simulink subsystem "MPC13_nlpsol"  (R2022b)
settings: Solver=VariableStepAuto  StartTime=0.0  StopTime=10.0  RelTol=1e-3
undefined symbols (not defined in the file): param_global, param_jointspace_ct, param_MPC10, param_MPC13, param_robot, param_traj, param_weight_init
settings Model: Creator=emu  LastModifiedBy=emu
settings OptimizationCC: ReuseModelBlockBuffer=on

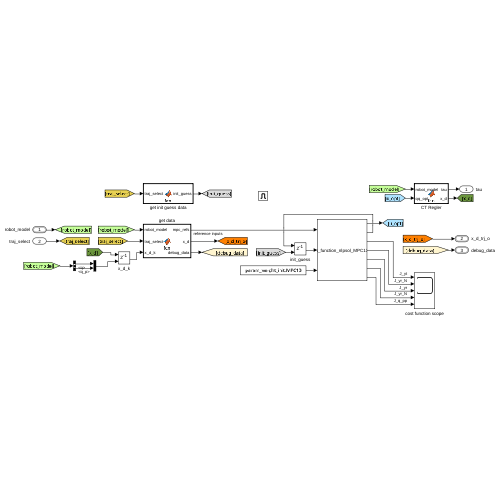
[thumbnail: Simulink's stored preview of the top-level diagram]
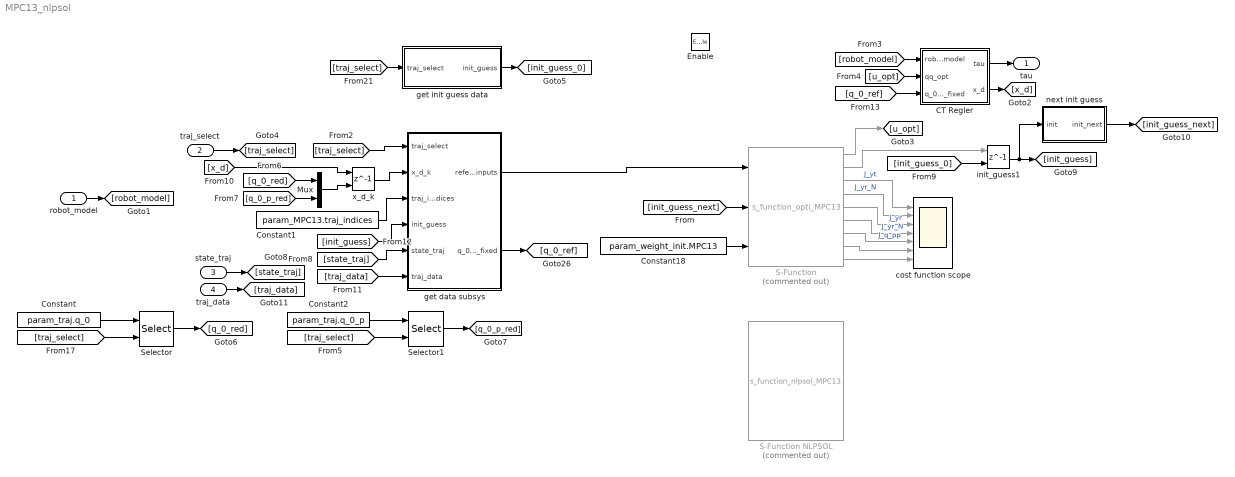
== system MPC13_nlpsol ==
  robot_model : Inport  OutDataTypeStr=Bus: robot_model
  traj_select : Inport  Port=2
  state_traj : Inport  Port=3  OutDataTypeStr=Bus: state_traj_bus
  traj_data : Inport  Port=4  OutDataTypeStr=Bus: traj_data_bus
  Enable : EnablePort
  CT Regler : MATLAB Function  TreatAsAtomicUnit=on
  Constant : Constant  Value=param_traj.q_0
  Constant1 : Constant  Value=param_MPC13.traj_indices
  Constant18 : Constant  Value=param_weight_init.MPC13  VectorParams1D=off
  Constant2 : Constant  Value=param_traj.q_0_p
  Mux : Mux  Inputs=2
  S-Function : S-Function  Commented=on  FunctionName=s_function_opti_MPC13  SFunctionModules='MPC13'  SFunctionDeploymentMode=off  EnableBusSupport=off
  S-Function NLPSOL : S-Function  Commented=on  FunctionName=s_function_nlpsol_MPC13  Parameters='s_functions/fr3_no_hand_6dof/MPC13.casadi', 'MPC13'  SFunctionModules='MPC13'  SFunctionDeploymentMode=off  EnableBusSupport=off
  Selector : Selector  NumberOfDimensions=2  InputPortWidth=3  IndexOptions=Index vector (dialog),Index vector (port)  Indices=param_robot.n_indices,1  OutputSizes=1,1
  Selector1 : Selector  NumberOfDimensions=2  InputPortWidth=3  IndexOptions=Index vector (dialog),Index vector (port)  Indices=param_robot.n_indices,1  OutputSizes=1,1
  cost function scope : Scope  NumInputPorts=7
  get data subsys : Subsystem
  get init guess data : MATLAB Function  TreatAsAtomicUnit=on
  init_guess1 : Delay  DelayLength=1  InitialConditionSource=Input port  InitialCondition=1  SampleTime=param_global.Ta
      settings: InputPortMap=u0,p4
  next init guess : MATLAB Function  TreatAsAtomicUnit=on
  x_d_k : Delay  DelayLength=1  InitialConditionSource=Input port  InitialCondition=1
      settings: InputPortMap=u0,p4
  tau : Outport
  wires:
  [init_guess_next] -> S-Function/2
  init_guess1/1 -> next init guess/1(init), [init_guess]
  next init guess/1(init_next) -> [init_guess_next]
  [state_traj] -> get data subsys/5(state_traj)
  S-Function/7 -> cost function scope/5  "J_q_pp"
  Mux/1 -> x_d_k/2
  [traj_select] -> get data subsys/1(traj_select)
  [robot_model] -> CT Regler/1(robot_model)
  Constant18/1 -> S-Function/3
  get data subsys/1(reference inputs) -> S-Function/1
  [q_0_p_red] -> Mux/2
  [traj_select] -> Selector1/2
  S-Function/8 -> cost function scope/6
  S-Function/6 -> cost function scope/4  "J_yr_N"
  [init_guess_0] -> init_guess1/2
  S-Function/5 -> cost function scope/3  "J_yr"
  get data subsys/2(q_0_ref_fixed) -> [q_0_ref]
  state_traj/1 -> [state_traj]
  [init_guess] -> get data subsys/4(init_guess)
  [q_0_red] -> Mux/1
  x_d_k/1 -> get data subsys/2(x_d_k)
  Selector/1 -> [q_0_red]
  [traj_select] -> get init guess data/1(traj_select)
  S-Function/1 -> [u_opt]
  [q_0_ref] -> CT Regler/3(q_0_ref_fixed)
  get init guess data/1(init_guess) -> [init_guess_0]
  robot_model/1 -> [robot_model]
  [traj_select] -> Selector/2
  Constant/1 -> Selector/1
  Constant2/1 -> Selector1/1
  Selector1/1 -> [q_0_p_red]
  [x_d] -> x_d_k/1
  CT Regler/1(tau) -> tau/1
  S-Function/9 -> cost function scope/7
  S-Function/4 -> cost function scope/2  "J_yr_N"
  S-Function/2 -> init_guess1/1
  Constant1/1 -> get data subsys/3(traj_indices)
  [u_opt] -> CT Regler/2(qq_opt)
  traj_select/1 -> [traj_select]
  S-Function/3 -> cost function scope/1  "J_yt"
  CT Regler/2(x_d) -> [x_d]
  traj_data/1 -> [traj_data]
  [traj_data] -> get data subsys/6(traj_data)

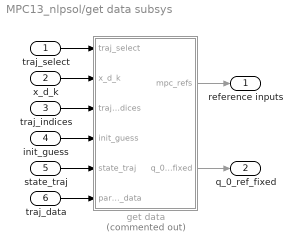
== system MPC13_nlpsol/get data subsys ==
  traj_select : Inport
  x_d_k : Inport  Port=2
  traj_indices : Inport  Port=3
  init_guess : Inport  Port=4
  state_traj : Inport  Port=5  OutDataTypeStr=Bus: state_traj_bus
  traj_data : Inport  Port=6  OutDataTypeStr=Bus: traj_data_bus
  get data : MATLAB Function  Commented=on  TreatAsAtomicUnit=on
  reference inputs : Outport
  q_0_ref_fixed : Outport  Port=2
  wires:
  traj_data/1 -> get data/6(param_traj_data)
  state_traj/1 -> get data/5(state_traj)
  traj_indices/1 -> get data/3(traj_indices)
  x_d_k/1 -> get data/2(x_d_k)
  get data/1(mpc_refs) -> reference inputs/1
  traj_select/1 -> get data/1(traj_select)
  init_guess/1 -> get data/4(init_guess)
  get data/2(q_0_ref_fixed) -> q_0_ref_fixed/1

== matlab function MPC13_nlpsol/CT Regler ==
  data: robot_model input Bus: robot_model; tau output; qq_opt input; q_0_ref_fixed input; param_robot parameter; param_jointspace_ct parameter; x_d output
function [tau, x_d] = fcn(robot_model, qq_opt, q_0_ref_fixed, param_robot, param_jointspace_ct)

n_indices = param_robot.n_indices;

n_red = param_robot.n_red;
n = param_robot.n_DOF;
q = robot_model.q;      % generalized coordinates
q_p = robot_model.q_p;  % time derivative of generalized coordinates

if size(qq_opt, 2) ~= 0 && size(qq_opt, 1) ~= 1
    n_indices_fixed = param_robot.n_indices_fixed;

    M = robot_model.M;      % inertia matrix
    g = robot_model.g;
    C_rnea = robot_model.C_rnea; % C_rnea(q, q_p) = C(q, q_p)q_p + g(q) = n(q, q_p)

    q_d_0_red    = qq_opt(1+0*n_red:1*n_red, 1); % q_0
    q_d_0_p_red  = qq_opt(1+1*n_red:2*n_red, 1); %q_p_0
    q_d_0_pp_red = qq_opt(1+2*n_red:3*n_red, 1); %q_p_00

    q_d_1_red    = qq_opt(1+3*n_red:4*n_red, 1); % q_1
    q_d_1_p_red  = qq_opt(1+4*n_red:5*n_red, 1); %q_p_1
    %q_d_1_pp_red = qq_opt(1+5*n_red:6*n_red, 1); %q_p_1

    q_d = zeros(n,1);
    q_d_p = zeros(n,1);
    q_d_pp = zeros(n,1);

    q_d(n_indices) = q_d_0_red;
    q_d(n_indices_fixed) = q_0_ref_fixed(n_indices_fixed);
    q_d_p(n_indices) = q_d_0_p_red;
    q_d_pp(n_indices) = q_d_0_pp_red;

    e = q - q_d;
    e_p = q_p - q_d_p;
    
    e(n_indices_fixed) = 0;
    e_p(n_indices_fixed) = 0;

    K_D_q = param_jointspace_ct.MPC12.K_D_q;
    K_P_q = param_jointspace_ct.MPC12.K_P_q;
    tau = M*(q_d_pp - K_D_q * e_p - K_P_q * e) + C_rnea - g;

    x_d = [q_d_1_red; q_d_1_p_red];
else
    tau = zeros(n,1);
    x_d = [q(n_indices); q_p(n_indices)];
end

== matlab function MPC13_nlpsol/get data subsys/get data ==
  settings: updateMethod=DISCRETE  sampleTime=param_global.Ta
  data: traj_select input; x_d_k input; traj_indices input; init_guess input; state_traj input Bus: state_traj_bus; mpc_refs output; param_robot parameter; param_traj parameter; q_0_ref_fixed output; param_traj_data input Bus: traj_data_bus
function [mpc_refs, q_0_ref_fixed] = fcn(traj_select, x_d_k, traj_indices, init_guess, state_traj, param_robot, param_traj, param_traj_data)
persistent cnt;
persistent run_flag;

if(isempty(cnt))
    cnt = 1;
    run_flag = 0;
end

n_red = param_robot.n_red;
traj_indices = traj_indices + (cnt-1);
N_MPC = length(traj_indices)-1;

% Parameters
x_k = x_d_k; % open loop mpc

% Assemble vector of recieved output measurements
p_d     = param_traj_data.p_d(   1:3, traj_indices, traj_select);
q_d     = param_traj_data.q_d(   1:4, traj_indices, traj_select);

y_d = [p_d; q_d];

%% Reference out
N_u = n_red*1;
N_q = n_red * (N_MPC+1);
q_k_prev = init_guess(1+N_u : N_u+N_q);
mpc_refs = [x_k(:); y_d(:); q_k_prev(:)]';

q_0_ref_fixed = param_traj.q_0(:, traj_select);

[run_flag, cnt] = update_traj_cnt(state_traj, run_flag, cnt, param_traj_data.N);

== matlab function MPC13_nlpsol/get init guess data ==
  data: traj_select input; param_MPC13_init_guess parameter; init_guess output
function init_guess   = fcn(traj_select, param_MPC13_init_guess)

init_guess = param_MPC13_init_guess.init_guess(traj_select,:);

== matlab function MPC13_nlpsol/next init guess ==
  data: init input; init_next output; param_MPC10 parameter; param_robot parameter; param_global parameter
function init_next = fcn(init, param_MPC10, param_robot, param_global)
param_MPC = param_MPC10;

Ta = param_global.Ta;
dt_arr = param_MPC.int_times;
N_MPC = param_MPC.N;
n_red = param_robot.n_red;
N_u = n_red * 1;
N_q = (n_red)*(N_MPC+1);

N = 0;

u_idx = N + [1:N_u];       N = N + length(u_idx);
q_idx = N + [1:N_q];       N = N + length(q_idx);
q_idx_2d = reshape(q_idx, n_red, (N_MPC+1));
q_idx_2d(:, 1:end-1) = q_idx_2d(:, 2:end);

q_init = init(q_idx_2d);

dq = (q_init(:, 2:end) - q_init(:, 1:end-1))./dt_arr;
q_next = q_init(:, 1:end-1) + dq * Ta;

x_idx_m1 = q_idx_2d(:, 1:end-1);

init_next = init';
init_next(x_idx_m1) = q_next;
